simulink model "check_control"  (R2015a)
settings: Solver=ode45  StartTime=0.0  StopTime=10.0  RelTol=1e-3
values from neighbouring files (symbols this model uses):
  A = [0 1; -1 -0.1]    [Q2C.m]
  B = [0;1]    [Q2C.m]
  C = [1 0]    [Q2C.m]
  D = 0    [Q2C.m]
libraries: simulink x1
settings Model: Creator=nightstalker  LastModifiedBy=nightstalker

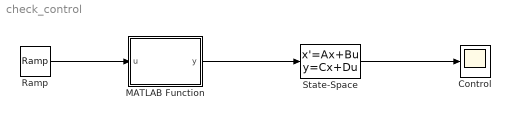
== system check_control ==
  Control : Scope
  MATLAB Function : MATLAB Function  TreatAsAtomicUnit=on
  Ramp : simulink/Sources/Ramp  slope=1  start=0  X0=0
  State-Space : StateSpace  A=A  B=B  C=C  D=D  X0=[1,0]
  wires:
  Ramp/1 -> MATLAB Function/1(u)
  MATLAB Function/1(y) -> State-Space/1
  State-Space/1 -> Control/1

== matlab function check_control/MATLAB Function ==
  data: u input; y output
function y = control_law(u)
U =  (1071925570109499860*cos(399^(1/2)*(u/20 - 1/2))*exp(u/20 + 1/2) + 92415637195996507*cos(399^(1/2)*(u/20 + 1/2))*exp(u/20 + 1/2) - 1164341207305496367*cos(399^(1/2)*(u/20 - 1/2))*exp(u/20 + 3/2) + 95333785585233340*399^(1/2)*exp(u/20 + 1/2)*sin(399^(1/2)*(u/20 - 1/2)) + 2918148389236833*399^(1/2)*exp(u/20 + 1/2)*sin(399^(1/2)*(u/20 + 1/2)) - 98251933974470173*399^(1/2)*exp(u/20 + 3/2)*sin(399^(1/2)*(u/20 - 1/2)))/(45035996273704960*(399*exp(2) - 800*exp(1) + 2*exp(1)*cos(399^(1/2)) + 399)), -(3696625487839860140*cos(399^(1/2)*(u/20 - 1/2))*exp(u/20 + 1/2) - 125675684450149307*cos(399^(1/2)*(u/20 + 1/2))*exp(u/20 + 1/2) - 3570949803389710833*cos(399^(1/2)*(u/20 - 1/2))*exp(u/20 + 3/2) - 116725935569473340*399^(1/2)*exp(u/20 + 1/2)*sin(399^(1/2)*(u/20 - 1/2)) + 8949748880675967*399^(1/2)*exp(u/20 + 1/2)*sin(399^(1/2)*(u/20 + 1/2)) + 107776186688797373*399^(1/2)*exp(u/20 + 3/2)*sin(399^(1/2)*(u/20 - 1/2)))/(90071992547409920*(399*exp(2) - 800*exp(1) + 2*exp(1)*cos(399^(1/2)) + 399));
y = U;
